simulink model "Mod5_Counter"  (R2020b)
settings: Solver=VariableStepAuto  StartTime=0.0  StopTime=10.0  RelTol=1e-3
libraries: simulink_extras x1
settings Model: Creator=shubham sharma  LastModifiedBy=shubham sharma

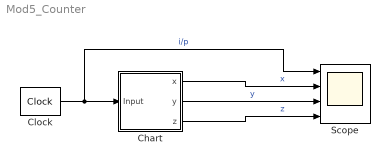
== system Mod5_Counter ==
  Chart : Stateflow chart  TreatAsAtomicUnit=on
  Clock : simulink_extras/Flip Flops/Clock  period=2
  Scope : Scope  NumInputPorts=4
  wires:
  Chart/1(x) -> Scope/2  "x"
  Chart/3(z) -> Scope/4  "z"
  Chart/2(y) -> Scope/3  "y"
  Clock/1 -> Scope/1, Chart/1(Input)  "i/p"

== stateflow chart Mod5_Counter/Chart ==
  state State1
    en: x=0; y=0; z=0;
  state State2
    en: z=0; y=0; x=1;
  state State3
    en: z=0;  y=1; x=0;
  state State4
    en: z=0; y=1;  x=1;
  state State5
    en: z=1; y=1; x=0;
  State5 -> State1 : {{z==1&&y==0&&x==0}}
  State4 -> State5 : {{z==0&&y==1&&x==1}}
  (default) -> State1
  State2 -> State3 : {{z==0&&y==0&&x==1}}
  State3 -> State4 : {{z==0&&y==1&&x==0}}
  State1 -> State2 : {z==0&&y==0&&x==0}
  data: x output; y output; z output; Input input
